simulink model "bh_1dof_compare_models"  (R2017a)
settings: Solver=ode15s  StartTime=0.0  StopTime=20  MaxStep=0.01  RelTol=1e-3  EnableMultiTasking=on
PreLoadFcn:
  | bh_script_1dof_params
values from neighbouring files (symbols this model uses):
  c = 2*0.2*3    (= 1.2)    [bh_script_1dof_params.m]
  k = 9    [bh_script_1dof_params.m]
  m = 1    [bh_script_1dof_params.m]
  x0 = 1    [bh_script_1dof_params.m]
  xdot_0 = 0    [bh_script_1dof_params.m]
libraries: fl_lib x8, nesl_utility x3
Description:
  | Copyright 2014 The MathWorks, Inc.
settings Model: Creator=smiller  LastModifiedBy=bhorton
settings DataIOCC: LimitDataPoints=on  SaveFormat=Array
settings OptimizationCC: LifeSpan=inf
settings DebuggingCC: UnderspecifiedInitializationDetection=Classic  MergeDetectMultiDrivingBlocksExec=none  SolverPrmCheckMsg=warning  AllowSymbolicDim=off  StateNameClashWarn=warning  SFUnexpectedBacktrackingDiag=warning  SFNoUnconditionalDefaultTransitionDiag=warning  SFExecutionAtInitializationDiag=none
settings HardwareCC: ProdBitPerPointer=32  ProdBitPerSizeT=32  ProdBitPerPtrDiffT=32  ProdLargestAtomicFloat=None  ProdIntDivRoundTo=Undefined  ProdEndianess=Unspecified  ProdWordSize=32  ProdHWDeviceType=32-bit Generic
settings ModelReferenceCC: PropagateSignalLabelsOutOfModel=off
settings GRTTargetCC: TargetLangStandard=C89/C90 (ANSI)  GeneratePreprocessorConditionals=Disable all
settings ConfigComp: CovMetricSettings=dw  CovHtmlReporting=on  CovSaveCumulativeToWorkspaceVar=on  CovSaveSingleToWorkspaceVar=on  CovExternalEMLEnable=off  CovSFcnEnable=off

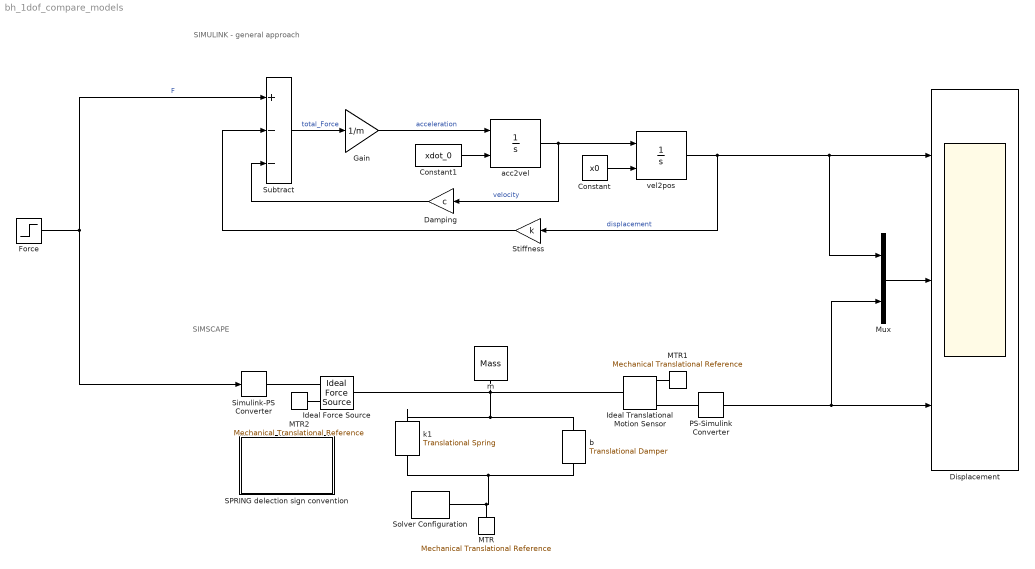
== system bh_1dof_compare_models ==
  note: SIMSCAPE
  note: SIMULINK - general approach
  Constant : Constant  Value=x0
  Constant1 : Constant  Value=xdot_0
  Damping : Gain  Gain=c
  Displacement : Scope  NumInputPorts=3
  Force : Step  Time=15  After=3  SampleTime=0
  Gain : Gain  Gain=1/m
  Ideal Force Source : fl_lib/Mechanical/Mechanical Sources/Ideal Force Source
  Ideal Translational Motion Sensor : fl_lib/Mechanical/Mechanical Sensors/Ideal Translational Motion Sensor  offset=def_k.xC m
      settings: AttributesFormatString=init POS = %<offset>
  MTR : fl_lib/Mechanical/Translational Elements/Mechanical Translational Reference
  MTR1 : fl_lib/Mechanical/Translational Elements/Mechanical Translational Reference
  MTR2 : fl_lib/Mechanical/Translational Elements/Mechanical Translational Reference
  Mux : Mux  Inputs=2
  PS-Simulink Converter : nesl_utility/PS-Simulink Converter  PhysicalDomain=network_engine_domain  SubClassName=ps_output  LeftPortType=input  RightPortType=output  PseudoPeriodic=off  Frequencies=[]  Unit=m  AffineConversion=off
  SPRING delection sign convention : Subsystem
  Simulink-PS Converter : nesl_utility/Simulink-PS Converter  PhysicalDomain=network_engine_domain  SubClassName=ps_input  LeftPortType=input  RightPortType=output  PseudoPeriodic=off  Frequencies=[]  NoiseDistribution=none  NoiseParameters=[]  Unit=N  AffineConversion=off  FilteringAndDerivatives=zero  SimscapeFilterOrder=1  InputFilterTimeConstant=.001  UdotUserProvided=0
  Solver Configuration : nesl_utility/Solver Configuration  PhysicalDomain=network_engine_domain  SubClassName=solver  LeftPortType=input  RightPortType=generic  Accelerate=off  Tones=[]  Harmonics=[]  SimulateNoise=off  Profile=off  UseLocalSampling=off  EnableSwitchedLinearOptims=on  FrequencyDomain=off  UseCCode=off  RelTol=0.001  AbsTol=1e-06  MinStep=1e-09  ToWorkspace=off  RevertToSquareIcSolve=off  NumHomotopyIterations=100  PhasorMode=off  PhasorModeNumHarmonics=1  OverrideAbsTol=off  DoDC=off  ResidualTolerance=1e-9  UseLocalSolver=off  LocalSolverChoice=NE_BACKWARD_EULER_ADVANCER  LocalSolverSampleTime=.001  DoFixedCost=off  MaxNonlinIter=12  MaxModeIter=2  LinearAlgebra=Sparse  DelaysMemoryBudget=1024  AutomaticFiltering=on  FilteringTimeConstant=0.001
  Stiffness : Gain  Gain=k
  Subtract : Sum  Inputs=+--
  acc2vel : Integrator  InitialConditionSource=external
  b : fl_lib/Mechanical/Translational Elements/Translational Damper  D=c N/(m/s)  v_specify=off  v_priority=None  v=0 m/s  v_nominal_specify=off  v_nominal_unit=m/s  v_nominal_value=1  f_specify=off  f_priority=None  f=0 N  f_nominal_specify=off  f_nominal_unit=N  f_nominal_value=1
  k1 : fl_lib/Mechanical/Translational Elements/Translational Spring  spr_rate=k N/m  v_specify=off  v_priority=High  v=xdot_0 m/s  v_nominal_specify=off  v_nominal_unit=m/s  v_nominal_value=1  f_specify=off  f_priority=None  f=0 N  f_nominal_specify=off  f_nominal_unit=N  f_nominal_value=1  x_specify=on  x_priority=High  x=def_k.x_def m  x_nominal_specify=off  x_nominal_unit=m  x_nominal_value=1
      settings: AttributesFormatString=DEF_X = %<x>
  m : fl_lib/Mechanical/Translational Elements/Mass  mass=m kg  v_specify=on  v_priority=None  v=def_k.vC m/s  v_nominal_specify=off  v_nominal_unit=m/s  v_nominal_value=1  f_specify=off  f_priority=None  f=0 N  f_nominal_specify=off  f_nominal_unit=N  f_nominal_value=1
      settings: AttributesFormatString=V0 = %<v>
  vel2pos : Integrator  InitialConditionSource=external
  wires:
  Subtract/1 -> Gain/1  "total_Force"
  Gain/1 -> acc2vel/1  "acceleration"
  vel2pos/1 -> Stiffness/1, Mux/1, Displacement/1  "displacement"
  Stiffness/1 -> Subtract/2
  Force/1 -> Simulink-PS Converter/1, Subtract/1  "F"
  Constant1/1 -> acc2vel/2
  acc2vel/1 -> vel2pos/1, Damping/1  "velocity"
  Damping/1 -> Subtract/3
  Constant/1 -> vel2pos/2
  PS-Simulink Converter/1 -> Mux/2, Displacement/3
  Mux/1 -> Displacement/2
  connections:
  k1/RConn1 -- b/RConn1 -- m/LConn1 -- Ideal Translational Motion Sensor/LConn1 -- Ideal Force Source/LConn1
  k1/LConn1 -- Solver Configuration/RConn1 -- MTR/LConn1 -- b/LConn1
  MTR2/LConn1 -- Ideal Force Source/RConn2
  Ideal Translational Motion Sensor/RConn3 -- PS-Simulink Converter/LConn1
  MTR1/LConn1 -- Ideal Translational Motion Sensor/RConn1
  Simulink-PS Converter/RConn1 -- Ideal Force Source/RConn1

== system bh_1dof_compare_models/SPRING delection sign convention ==
  note: deflection is NEGATIVE (-)
  note: deflection is POSITIVE (+)
  note: Recall the definition of deflection:
      |
      |          DEF = X_R - X_C
